simulink model "sd_task_new"  (Simulink 8.4)
settings: Solver=ode3  StartTime=0.0  StopTime=t(end)  FixedStep=t(2)-t(1)  RelTol=1e-3
undefined symbols (not defined in the file or in its folder): pp, ptf
settings Model: Creator=Frank Drop  LastModifiedBy=fmdrop  CovHtmlReporting=off
settings DataIOCC: ExternalInput=[iS, t, ptf_Ypt, ptf_Ype, ptf_Ynms, ptf_Yc, tp, pp]
settings OptimizationCC: AccelVerboseBuild=on
settings DebuggingCC: ArrayBoundsChecking=warning
settings SFSimCC: SFSimEnableDebug=off

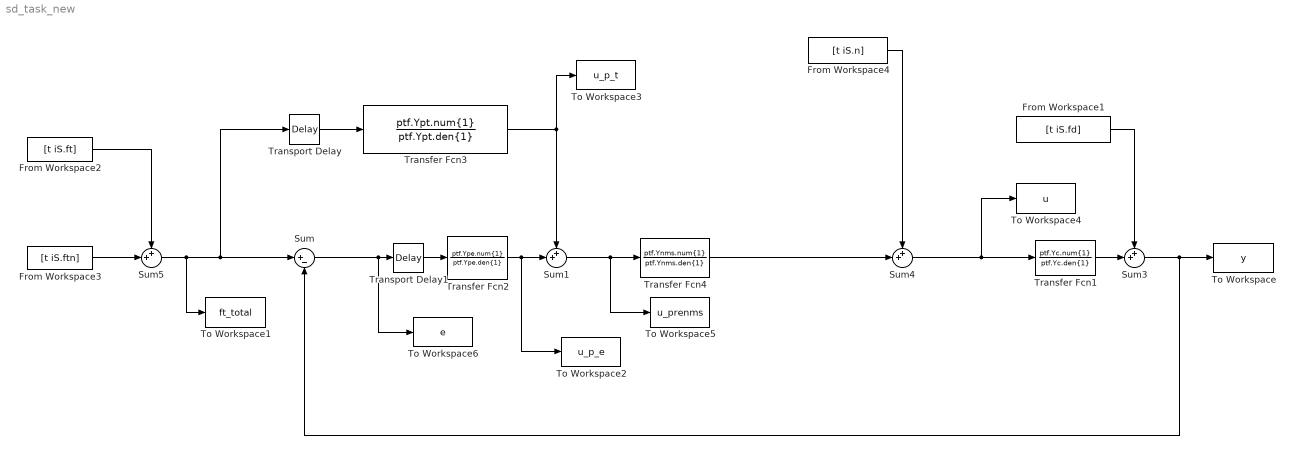
== system sd_task_new ==
  From Workspace1 : FromWorkspace  VariableName=[t iS.fd]  SampleTime=0
  From Workspace2 : FromWorkspace  VariableName=[t iS.ft]  SampleTime=0
  From Workspace3 : FromWorkspace  VariableName=[t iS.ftn]  SampleTime=0
  From Workspace4 : FromWorkspace  VariableName=[t iS.n]  SampleTime=0
  Sum : Sum  Inputs=|+-
  Sum{1,3..5} (4 alike) : Sum  Inputs=++|
  To Workspace : ToWorkspace  VariableName=y  SampleTime=-1
  To Workspace1 : ToWorkspace  VariableName=ft_total  SampleTime=-1
  To Workspace2 : ToWorkspace  VariableName=u_p_e  SampleTime=-1
  To Workspace3 : ToWorkspace  VariableName=u_p_t  SampleTime=-1
  To Workspace4 : ToWorkspace  VariableName=u  SampleTime=-1
  To Workspace5 : ToWorkspace  VariableName=u_prenms  SampleTime=-1
  To Workspace6 : ToWorkspace  VariableName=e  SampleTime=-1
  Transfer Fcn1 : TransferFcn  Numerator=ptf.Yc.num{1}  Denominator=ptf.Yc.den{1}
  Transfer Fcn2 : TransferFcn  Numerator=ptf.Ype.num{1}  Denominator=ptf.Ype.den{1}
  Transfer Fcn3 : TransferFcn  Numerator=ptf.Ypt.num{1}  Denominator=ptf.Ypt.den{1}
  Transfer Fcn4 : TransferFcn  Numerator=ptf.Ynms.num{1}  Denominator=ptf.Ynms.den{1}
  Transport Delay : TransportDelay  DelayTime=pp.tau_p_t
  Transport Delay1 : TransportDelay  DelayTime=pp.tau_p_e
  wires:
  Transport Delay/1 -> Transfer Fcn3/1
  Sum/1 -> Transport Delay1/1, To Workspace6/1
  Transport Delay1/1 -> Transfer Fcn2/1
  Sum1/1 -> To Workspace5/1, Transfer Fcn4/1
  Transfer Fcn1/1 -> Sum3/2
  From Workspace1/1 -> Sum3/1
  Sum4/1 -> Transfer Fcn1/1, To Workspace4/1
  From Workspace4/1 -> Sum4/1
  Transfer Fcn3/1 -> To Workspace3/1, Sum1/1
  Transfer Fcn2/1 -> Sum1/2, To Workspace2/1
  Sum3/1 -> To Workspace/1, Sum/2
  Transfer Fcn4/1 -> Sum4/2
  From Workspace3/1 -> Sum5/2
  From Workspace2/1 -> Sum5/1
  Sum5/1 -> Sum/1, Transport Delay/1, To Workspace1/1
